simulink library "casper_library_ffts"  (R2021a)
settings: Solver=ode45  StartTime=0.0  StopTime=10.0  RelTol=1e-3
(part 2 of 2)

== system casper_library_ffts/fft_wideband_real ==
